simulink model "Amplitude_modulation_exp_2"  (R2021a)
settings: Solver=VariableStepAuto  StartTime=0.0  StopTime=10.0  RelTol=1e-3
libraries: dsparch4 x1
settings Model: Creator=Devraj Kashyap  LastModifiedBy=ritav

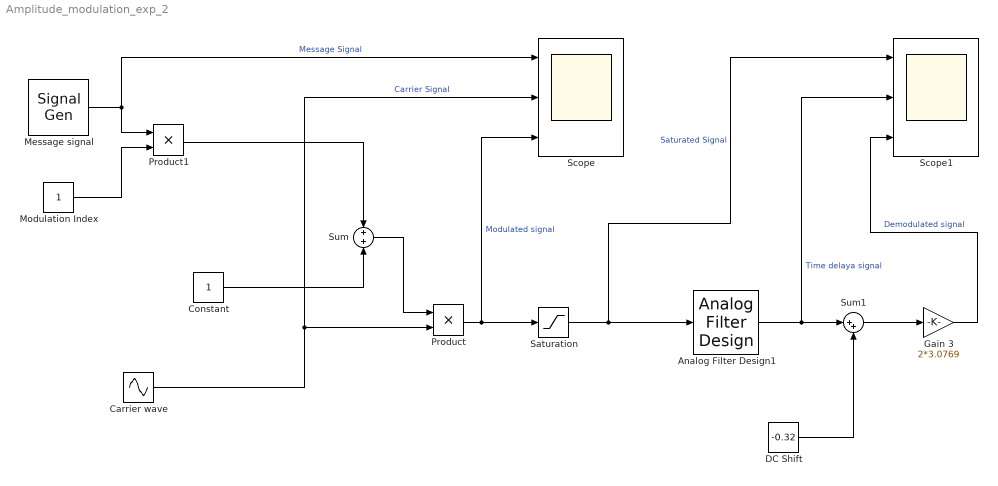
== system Amplitude_modulation_exp_2 ==
  Analog Filter Design1 : dsparch4/Analog Filter Design  method=Butterworth  filttype=Lowpass  N=9  Wlo=100  Whi=80  Rp=2  Rs=40
  Carrier wave : Sin  Frequency=2*pi*75  SampleTime=.001
  Constant : Constant
  DC Shift : Constant  Value=-0.32
  Gain 3 : Gain  Gain=2*3.0769
  Message signal : SignalGenerator  Frequency=2*pi*5  Units=rad/sec
  Modulation Index : Constant
  Product : Product  RndMeth=Ceiling
  Product1 : Product
  Saturation : Saturate  UpperLimit=5  LowerLimit=0
  Scope : Scope  NumInputPorts=3
  Scope1 : Scope  NumInputPorts=3
  Sum : Sum  RndMeth=Ceiling
  Sum1 : Sum  Inputs=|++
  wires:
  Constant/1 -> Sum/2
  Sum/1 -> Product/1
  Carrier wave/1 -> Scope/2, Product/2  "Carrier Signal"
  Product/1 -> Saturation/1, Scope/3  "Modulated signal"
  Message signal/1 -> Scope/1, Product1/1  "Message Signal"
  Modulation Index/1 -> Product1/2
  Product1/1 -> Sum/1
  Saturation/1 -> Scope1/1, Analog Filter Design1/1  "Saturated Signal"
  Analog Filter Design1/1 -> Sum1/1, Scope1/2  "Time delaya signal"
  DC Shift/1 -> Sum1/2
  Sum1/1 -> Gain 3/1
  Gain 3/1 -> Scope1/3  "Demodulated signal"
